simulink subsystem "controller"  (R2026a)
settings: Solver=VariableStepAuto
settings Model: DataDictionary=controllerParams.sldd  EnableAccessToBaseWorkspace=off  Creator=maxhu  LastModifiedBy=maxhu

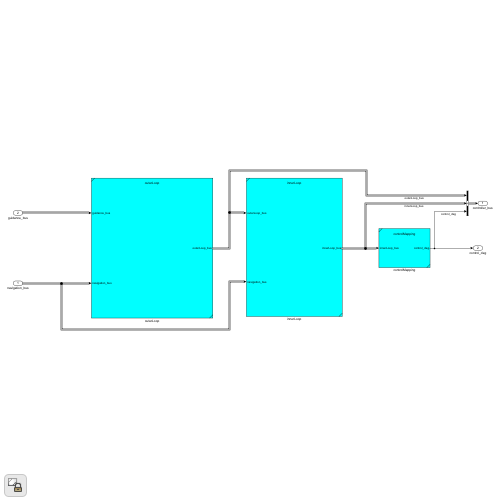
[thumbnail: Simulink's stored preview of the top-level diagram]
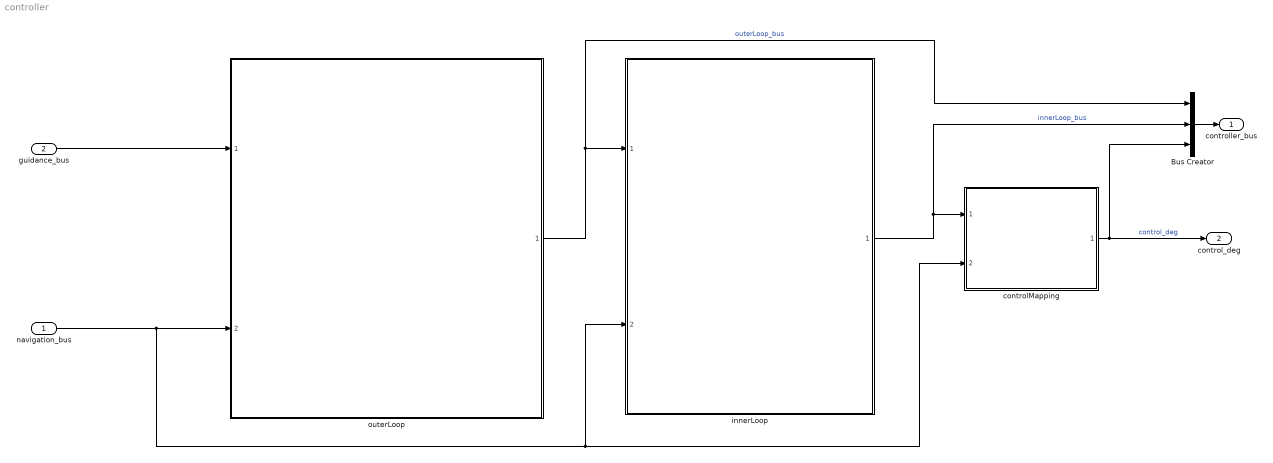
== system controller ==
  navigation_bus : Inport
  guidance_bus : Inport  Port=2
  Bus Creator : BusCreator  Inputs=3
  controlMapping : Subsystem  ReferencedSubsystem=controlMapping
  innerLoop : Subsystem  ReferencedSubsystem=innerLoop
  outerLoop : Subsystem  ReferencedSubsystem=outerLoop
  controller_bus : Outport
  control_deg : Outport  Port=2
  wires:
  controlMapping/1 -> control_deg/1, Bus Creator/3  "control_deg"
  innerLoop/1 -> controlMapping/1, Bus Creator/2  "innerLoop_bus"
  outerLoop/1 -> Bus Creator/1, innerLoop/1  "outerLoop_bus"
  navigation_bus/1 -> outerLoop/2, innerLoop/2, controlMapping/2
  guidance_bus/1 -> outerLoop/1
  Bus Creator/1 -> controller_bus/1
